simulink model "chuanbiquxian"  (Simulink 7.4)
settings: Solver=ode45  StartTime=0.0  StopTime=30000  RelTol=1e-3
libraries: simulink x1
settings Model: Creator=admini  LastModifiedBy=admini

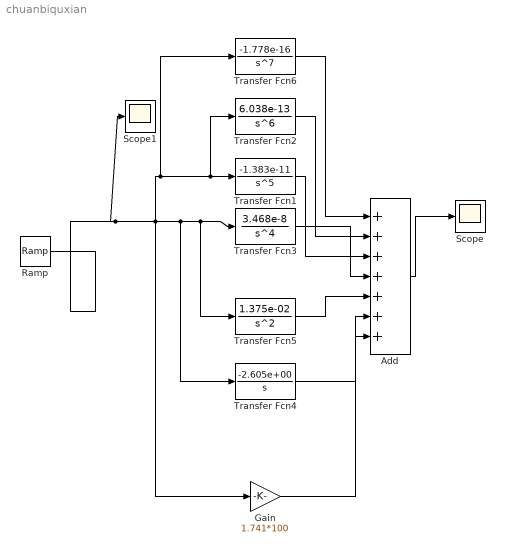
== system chuanbiquxian ==
  Add : Sum  Inputs=+++++++  OutDataType=fixdt(1, 16)  OutScaling=2^-10
  Gain : Gain  Gain=1.741*100  ParameterDataType=fixdt(1, 16)  ParameterScaling=2^0  OutDataType=fixdt(1, 16)  OutScaling=2^0
  Ramp : simulink/Sources/Ramp  SystemSampleTime=-1  slope=1  start=0  X0=0
  Scope : Scope
      settings: TimeRange=10000  YMin=-2000000000  YMax=12000000000
  Scope1 : Scope
  Transfer Fcn1 : TransferFcn  Numerator=[-1.383e-11]  Denominator=[1 0 0 0 0 0]
  Transfer Fcn2 : TransferFcn  Numerator=[ 6.038e-13]  Denominator=[1 0 0 0 0 0 0]
  Transfer Fcn3 : TransferFcn  Numerator=[3.468e-8]  Denominator=[1 0 0 0 0]
  Transfer Fcn4 : TransferFcn  Numerator=[-2.605e+00]  Denominator="[1  0]"
  Transfer Fcn5 : TransferFcn  Numerator=[ 1.375e-02]  Denominator="[1  0 0]"
  Transfer Fcn6 : TransferFcn  Numerator=[ -1.778e-16]  Denominator=[1 0 0 0 0 0 0 0]
  wires:
  Add/1 -> Scope/1
  Ramp/1 -> Gain/1, Transfer Fcn3/1, Transfer Fcn5/1, Transfer Fcn4/1, Transfer Fcn6/1, Transfer Fcn1/1, Transfer Fcn2/1, Scope1/1
  Transfer Fcn6/1 -> Add/1
  Transfer Fcn2/1 -> Add/2
  Transfer Fcn1/1 -> Add/3
  Transfer Fcn3/1 -> Add/4
  Transfer Fcn5/1 -> Add/5
  Transfer Fcn4/1 -> Add/6
  Gain/1 -> Add/7
